simulink model "meat_1024pt_bee2_sign"  (Simulink 6.2)
settings: Solver=ode45  StartTime=0.0  StopTime=60000  RelTol=1e-3
undefined symbols (not defined in the file): BEE2_usr, bit_rev, pfb_coeff_gen_calc
libraries: xbsIndex_r3 x1079, casper_library x94, xps_library x27
(part 2 of 8)

== system meat_1024pt_bee2_sign/fft ==
  sync : Inport  Port=1  LatchInput=off
  shift : Inport  Port=2  LatchInput=off
  pol0 : Inport  Port=3  LatchInput=off
  pol1 : Inport  Port=4  LatchInput=off
  fft_biplex0 : Subsystem  AncestorBlock=casper_library/FFTs/fft_biplex  mask(fft_biplex){FFTSize=10, BitWidth=18, quantization=Truncate, overflow=Wrap, add_latency=3, mult_latency=4, bram_latency=3}
      mask prompts: FFTSize "Size of FFT: (2^? pnts)"; BitWidth "Bitwidth: (Max Efficiency at 18 bits)"; quantization "Quantization Behavior"; overflow "Overflow Behavior"; add_latency "Add Latency"; mult_latency "Mult Latency"; bram_latency "BRAM Latency"
      mask init:
      | fft_biplex_init(gcb,...
      |     'FFTSize', FFTSize,...
      |     'BitWidth', BitWidth,...
      |     'quantization', quantization,...
      |     'overflow', overflow,...
      |     'add_latency', add_latency,...
      |     'mult_latency', mult_latency,...
      |     'bram_latency', bram_latency);
      settings: AttributesFormatString=FFTSize=10, BitWidth=18
      mask StyleString: edit,edit,popup(Truncate|Round  (unbiased: +/- Inf)|Round  (unbiased: Even Values)),popup(Wrap|Saturate|Error),edit,edit,edit
  sync_out : Outport
  out0 : Outport  Port=2
  out1 : Outport  Port=3
  wires:
  pol0/1 -> fft_biplex0/1(pol1)
  pol1/1 -> fft_biplex0/2(pol2)
  shift/1 -> fft_biplex0/4(shift)
  sync/1 -> fft_biplex0/3(sync)
  fft_biplex0/1(pol1_out) -> out0/1
  fft_biplex0/2(pol2_out) -> out1/1
  fft_biplex0/4(sync_out) -> sync_out/1

== system meat_1024pt_bee2_sign/pfb_fir ==
  sync : Inport  Port=1  LatchInput=off
  pol1_in1 : Inport  Port=2  LatchInput=off
  pol2_in1 : Inport  Port=3  LatchInput=off
  pol1_in1_first_tap : Subsystem  AncestorBlock=casper_library/PFBs/first_tap  mask(first_tap){nput=0, PFBSize=10, CoeffBitWidth=8, TotalTaps=4, BitWidthIn=8, CoeffDistMem=1, WindowType=hamming, mult_latency=3, bram_latency=3, n_inputs=0, fwidth=1}
      mask prompts: nput "This is input number:"; PFBSize "Size of PFB: (2^? pnts)"; CoeffBitWidth "Bitwidth of Coefficients:"; TotalTaps "Total Number of Taps:"; BitWidthIn "Input Bitwidth:"; CoeffDistMem "Implement Coeff Gen in Distributed Memory:"; WindowType "Windowing Function:"; mult_latency "Mult Latency"; bram_latency "BRAM Latency"; n_inputs "Number of Simultaneous Inputs: (2^?)"; fwidth "Bit Width (normal=1)"
      mask init:
      | first_tap_init(gcb,...
      |     'nput', nput,...
      |     'PFBSize', PFBSize,...
      |     'CoeffBitWidth', CoeffBitWidth,...
      |     'TotalTaps', TotalTaps,...
      |     'BitWidthIn', BitWidthIn,...
      |     'CoeffDistMem', CoeffDistMem,...
      |     'WindowType', WindowType,...
      |     'mult_latency', mult_latency,...
      |     'bram_latency', bram_latency,...
      |     'n_inputs', n_inputs,...
      |     'fwidth', fwidth);
      settings: AttributesFormatString=input=0, taps=4
      mask StyleString: edit,edit,edit,edit,edit,edit,popup(bartlett|barthannwin|blackman|blackmanharris|bohamwin|chebwin|flattopwin|gausswin|hamming|hann|kaiser|nuttallwin|parzenwin|rectwin|tukeywin|triang),edit,edit,edit,edit
  pol1_in1_last_tap : Subsystem  AncestorBlock=casper_library/PFBs/last_tap  mask(last_tap){TotalTaps=4, BitWidthIn=8, BitWidthOut=18, CoeffBitWidth=8, add_latency=2, mult_latency=3, quantization=Truncate}
      mask prompts: TotalTaps "Total Number of Taps:"; BitWidthIn "Input Bitwidth:"; BitWidthOut "Output Bitwidth:"; CoeffBitWidth "Coeff Bitwidth:"; add_latency "Add Latency"; mult_latency "Mult Latency"; quantization "Quantization Behavior"
      mask init:
      | last_tap_init(gcb,...
      |     'TotalTaps', TotalTaps,...
      |     'BitWidthIn', BitWidthIn,...
      |     'BitWidthOut', BitWidthOut,...
      |     'CoeffBitWidth', CoeffBitWidth,...
      |     'add_latency', add_latency,...
      |     'mult_latency', mult_latency,...
      |     'quantization', quantization);
      settings: AttributesFormatString=taps=4
      mask StyleString: edit,edit,edit,edit,edit,edit,popup(Truncate|Round  (unbiased: +/- Inf)|Round  (unbiased: Even Values))
  pol1_in1_tap2 : casper_library/PFBs/tap
      link override delay/delay_bram/Constant2: equ=P=C
      link override sync_delay/Constant: equ=P=C
      link override sync_delay/Constant1: equ=P=C
      link override sync_delay/Constant2: equ=P=C
      link override sync_delay/Constant3: equ=P=C
  pol1_in1_tap3 : casper_library/PFBs/tap
      link override delay/delay_bram/Constant2: equ=P=C
      link override sync_delay/Constant: equ=P=C
      link override sync_delay/Constant1: equ=P=C
      link override sync_delay/Constant2: equ=P=C
      link override sync_delay/Constant3: equ=P=C
  pol2_in1_first_tap : Subsystem  AncestorBlock=casper_library/PFBs/first_tap  mask(first_tap){nput=0, PFBSize=10, CoeffBitWidth=8, TotalTaps=4, BitWidthIn=8, CoeffDistMem=1, WindowType=hamming, mult_latency=3, bram_latency=3, n_inputs=0, fwidth=1}
      mask prompts: nput "This is input number:"; PFBSize "Size of PFB: (2^? pnts)"; CoeffBitWidth "Bitwidth of Coefficients:"; TotalTaps "Total Number of Taps:"; BitWidthIn "Input Bitwidth:"; CoeffDistMem "Implement Coeff Gen in Distributed Memory:"; WindowType "Windowing Function:"; mult_latency "Mult Latency"; bram_latency "BRAM Latency"; n_inputs "Number of Simultaneous Inputs: (2^?)"; fwidth "Bit Width (normal=1)"
      mask init: same as meat_1024pt_bee2_sign/pfb_fir/pol1_in1_first_tap
      settings: AttributesFormatString=input=0, taps=4
      mask StyleString: edit,edit,edit,edit,edit,edit,popup(bartlett|barthannwin|blackman|blackmanharris|bohamwin|chebwin|flattopwin|gausswin|hamming|hann|kaiser|nuttallwin|parzenwin|rectwin|tukeywin|triang),edit,edit,edit,edit
  pol2_in1_last_tap : Subsystem  AncestorBlock=casper_library/PFBs/last_tap  mask(last_tap){TotalTaps=4, BitWidthIn=8, BitWidthOut=18, CoeffBitWidth=8, add_latency=2, mult_latency=3, quantization=Truncate}
      mask prompts: TotalTaps "Total Number of Taps:"; BitWidthIn "Input Bitwidth:"; BitWidthOut "Output Bitwidth:"; CoeffBitWidth "Coeff Bitwidth:"; add_latency "Add Latency"; mult_latency "Mult Latency"; quantization "Quantization Behavior"
      mask init: same as meat_1024pt_bee2_sign/pfb_fir/pol1_in1_last_tap
      settings: AttributesFormatString=taps=4
      mask StyleString: edit,edit,edit,edit,edit,edit,popup(Truncate|Round  (unbiased: +/- Inf)|Round  (unbiased: Even Values))
  pol2_in1_tap2 : casper_library/PFBs/tap
      link override delay/delay_bram/Constant2: equ=P=C
      link override sync_delay/Constant: equ=P=C
      link override sync_delay/Constant1: equ=P=C
      link override sync_delay/Constant2: equ=P=C
      link override sync_delay/Constant3: equ=P=C
  pol2_in1_tap3 : casper_library/PFBs/tap
      link override delay/delay_bram/Constant2: equ=P=C
      link override sync_delay/Constant: equ=P=C
      link override sync_delay/Constant1: equ=P=C
      link override sync_delay/Constant2: equ=P=C
      link override sync_delay/Constant3: equ=P=C
  sync_out : Outport
  pol1_out1 : Outport  Port=2
  pol2_out1 : Outport  Port=3
  wires:
  pol1_in1/1 -> pol1_in1_first_tap/1(din)
  sync/1 -> pol1_in1_first_tap/2(sync), pol2_in1_first_tap/2(sync)
  pol1_in1_first_tap/1(dout) -> pol1_in1_tap2/1
  pol1_in1_first_tap/2(sync_out) -> pol1_in1_tap2/2
  pol1_in1_first_tap/3(coeff_out) -> pol1_in1_tap2/3
  pol1_in1_first_tap/4(taps_out) -> pol1_in1_tap2/4
  pol1_in1_tap2/1 -> pol1_in1_tap3/1
  pol1_in1_tap2/2 -> pol1_in1_tap3/2
  pol1_in1_tap2/3 -> pol1_in1_tap3/3
  pol1_in1_tap2/4 -> pol1_in1_tap3/4
  pol1_in1_tap3/1 -> pol1_in1_last_tap/1(din)
  pol1_in1_tap3/2 -> pol1_in1_last_tap/2(sync)
  pol1_in1_tap3/3 -> pol1_in1_last_tap/3(coeff)
  pol1_in1_tap3/4 -> pol1_in1_last_tap/4(taps)
  pol1_in1_last_tap/1(dout) -> pol1_out1/1
  pol1_in1_last_tap/2(sync_out) -> sync_out/1
  pol2_in1/1 -> pol2_in1_first_tap/1(din)
  pol2_in1_first_tap/1(dout) -> pol2_in1_tap2/1
  pol2_in1_first_tap/2(sync_out) -> pol2_in1_tap2/2
  pol2_in1_first_tap/3(coeff_out) -> pol2_in1_tap2/3
  pol2_in1_first_tap/4(taps_out) -> pol2_in1_tap2/4
  pol2_in1_tap2/1 -> pol2_in1_tap3/1
  pol2_in1_tap2/2 -> pol2_in1_tap3/2
  pol2_in1_tap2/3 -> pol2_in1_tap3/3
  pol2_in1_tap2/4 -> pol2_in1_tap3/4
  pol2_in1_tap3/1 -> pol2_in1_last_tap/1(din)
  pol2_in1_tap3/2 -> pol2_in1_last_tap/2(sync)
  pol2_in1_tap3/3 -> pol2_in1_last_tap/3(coeff)
  pol2_in1_tap3/4 -> pol2_in1_last_tap/4(taps)
  pol2_in1_last_tap/1(dout) -> pol2_out1/1

== system meat_1024pt_bee2_sign/pol1_kurt1 ==
  note: Input unsigned 24-bits, b.p. at 23
  note: Output unsigned 24-bits, b.p. at 23
  note: Unsigned, 18-bits, b.p. at 12
  coeff : Inport  Orientation=down  Port=1  LatchInput=off
  data_in : Inport  Port=2  LatchInput=off
  Convert : xbsIndex_r3/Convert  arith_type=Unsigned  n_bits=32  bin_pt=31  quantization=Truncate  overflow=Wrap  latency=1  explicit_period=off  period=1  dbl_ovrd=off  show_param=off  inserted_by_tool=off  pipeline=off
      settings: xl_area=[0, 0, 0, 0, 0, 0, 0]
  mult_coeff_fft_real : xbsIndex_r3/Mult  precision=Full  arith_type="Signed  (2's comp)"  n_bits=24  bin_pt=23  quantization=Truncate  overflow=Wrap  latency=5  explicit_period=off  period=1  en=off  dbl_ovrd=off  show_param=on  mult_type=Parallel  oversample=2  use_embedded=on  pipeline=on  use_rpm=on  placement_style=Rectangular Shape  gen_core=off
      settings: xl_area=[0, 0, 0, 0, 0, 0, 0]
  data_out : Outport
  wires:
  Convert/1 -> data_out/1
  data_in/1 -> mult_coeff_fft_real/2
  coeff/1 -> mult_coeff_fft_real/1
  mult_coeff_fft_real/1 -> Convert/1

== system meat_1024pt_bee2_sign/pol2_kurt1 ==
  note: Unsigned, 18-bits, b.p. at 12
  note: Output unsigned 24-bits, b.p. at 23
  note: Input unsigned 24-bits, b.p. at 23
  coeff : Inport  Orientation=down  Port=1  LatchInput=off
  data_in : Inport  Port=2  LatchInput=off
  Convert : xbsIndex_r3/Convert  arith_type=Unsigned  n_bits=32  bin_pt=31  quantization=Truncate  overflow=Wrap  latency=1  explicit_period=off  period=1  dbl_ovrd=off  show_param=off  inserted_by_tool=off  pipeline=off
      settings: xl_area=[0, 0, 0, 0, 0, 0, 0]
  mult_coeff_fft_real : xbsIndex_r3/Mult  precision=Full  arith_type="Signed  (2's comp)"  n_bits=24  bin_pt=23  quantization=Truncate  overflow=Wrap  latency=5  explicit_period=off  period=1  en=off  dbl_ovrd=off  show_param=on  mult_type=Parallel  oversample=2  use_embedded=on  pipeline=on  use_rpm=on  placement_style=Rectangular Shape  gen_core=off
      settings: xl_area=[0, 0, 0, 0, 0, 0, 0]
  data_out : Outport
  wires:
  Convert/1 -> data_out/1
  mult_coeff_fft_real/1 -> Convert/1
  coeff/1 -> mult_coeff_fft_real/1
  data_in/1 -> mult_coeff_fft_real/2

== system meat_1024pt_bee2_sign/signed_bitselect ==
  bitselect : Inport  Port=1  LatchInput=off
  data_in : Inport  Port=2  LatchInput=off
  0-6_inclusive : xbsIndex_r3/Slice  mode=Lower Bit Location + Width  nbits=7  bit1=0  base1=MSB of Input  bit0=0  base0=LSB of Input  boolean_output=off  explicit_period=off  period=1  dbl_ovrd=off
  14-20_inclusive : xbsIndex_r3/Slice  mode=Lower Bit Location + Width  nbits=7  bit1=0  base1=MSB of Input  bit0=14  base0=LSB of Input  boolean_output=off  explicit_period=off  period=1  dbl_ovrd=off
  21-27_inclusive : xbsIndex_r3/Slice  mode=Lower Bit Location + Width  nbits=7  bit1=0  base1=MSB of Input  bit0=7  base0=LSB of Input  boolean_output=off  explicit_period=off  period=1  dbl_ovrd=off
  28-34_inclusive : xbsIndex_r3/Slice  mode=Lower Bit Location + Width  nbits=7  bit1=0  base1=MSB of Input  bit0=7  base0=LSB of Input  boolean_output=off  explicit_period=off  period=1  dbl_ovrd=off
  35-41_inclusive : xbsIndex_r3/Slice  mode=Lower Bit Location + Width  nbits=7  bit1=0  base1=MSB of Input  bit0=7  base0=LSB of Input  boolean_output=off  explicit_period=off  period=1  dbl_ovrd=off
  40-47_inclusive : xbsIndex_r3/Slice  mode=Lower Bit Location + Width  nbits=7  bit1=0  base1=MSB of Input  bit0=7  base0=LSB of Input  boolean_output=off  explicit_period=off  period=1  dbl_ovrd=off
  7-13_inclusive : xbsIndex_r3/Slice  mode=Lower Bit Location + Width  nbits=7  bit1=0  base1=MSB of Input  bit0=7  base0=LSB of Input  boolean_output=off  explicit_period=off  period=1  dbl_ovrd=off
  Concat{,1..5} (6 alike) : xbsIndex_r3/Concat  num_inputs=2  explicit_period=off  period=1  dbl_ovrd=off
  Mux : xbsIndex_r3/Mux  inputs=7  precision=Full  arith_type="Signed  (2's comp)"  n_bits=8  bin_pt=2  quantization=Truncate  overflow=Wrap  latency=0  explicit_period=off  period=1  en=off  dbl_ovrd=off  show_param=off  mux_type=off  use_rpm=off  gen_core=off
      settings: xl_area=[0, 0, 0, 0, 0, 0, 0]
  sign_bit : xbsIndex_r3/Slice  mode=Upper Bit Location + Width  nbits=1  bit1=0  base1=MSB of Input  bit0=0  base0=LSB of Input  boolean_output=off  explicit_period=off  period=1  dbl_ovrd=off
  data_out : Outport
  wires:
  Mux/1 -> data_out/1
  bitselect/1 -> Mux/1
  0-6_inclusive/1 -> Concat/2
  7-13_inclusive/1 -> Concat1/2
  14-20_inclusive/1 -> Concat2/2
  21-27_inclusive/1 -> Concat3/2
  28-34_inclusive/1 -> Concat4/2
  35-41_inclusive/1 -> Concat5/2
  sign_bit/1 -> Concat/1, Concat1/1, Concat2/1, Concat3/1, Concat4/1, Concat5/1
  data_in/1 -> sign_bit/1, 0-6_inclusive/1, 7-13_inclusive/1, 14-20_inclusive/1, 21-27_inclusive/1, 28-34_inclusive/1, 35-41_inclusive/1, 40-47_inclusive/1
  Concat/1 -> Mux/2
  Concat1/1 -> Mux/3
  Concat2/1 -> Mux/4
  Concat3/1 -> Mux/5
  Concat4/1 -> Mux/6
  Concat5/1 -> Mux/7
  40-47_inclusive/1 -> Mux/8

== system meat_1024pt_bee2_sign/signed_bitselect_1 ==
  bitselect : Inport  Port=1  LatchInput=off
  data_in : Inport  Port=2  LatchInput=off
  0-6_inclusive : xbsIndex_r3/Slice  mode=Lower Bit Location + Width  nbits=7  bit1=0  base1=MSB of Input  bit0=0  base0=LSB of Input  boolean_output=off  explicit_period=off  period=1  dbl_ovrd=off
  14-20_inclusive : xbsIndex_r3/Slice  mode=Lower Bit Location + Width  nbits=7  bit1=0  base1=MSB of Input  bit0=14  base0=LSB of Input  boolean_output=off  explicit_period=off  period=1  dbl_ovrd=off
  21-27_inclusive : xbsIndex_r3/Slice  mode=Lower Bit Location + Width  nbits=7  bit1=0  base1=MSB of Input  bit0=7  base0=LSB of Input  boolean_output=off  explicit_period=off  period=1  dbl_ovrd=off
  28-34_inclusive : xbsIndex_r3/Slice  mode=Lower Bit Location + Width  nbits=7  bit1=0  base1=MSB of Input  bit0=7  base0=LSB of Input  boolean_output=off  explicit_period=off  period=1  dbl_ovrd=off
  35-41_inclusive : xbsIndex_r3/Slice  mode=Lower Bit Location + Width  nbits=7  bit1=0  base1=MSB of Input  bit0=7  base0=LSB of Input  boolean_output=off  explicit_period=off  period=1  dbl_ovrd=off
  40-47_inclusive : xbsIndex_r3/Slice  mode=Lower Bit Location + Width  nbits=7  bit1=0  base1=MSB of Input  bit0=7  base0=LSB of Input  boolean_output=off  explicit_period=off  period=1  dbl_ovrd=off
  7-13_inclusive : xbsIndex_r3/Slice  mode=Lower Bit Location + Width  nbits=7  bit1=0  base1=MSB of Input  bit0=7  base0=LSB of Input  boolean_output=off  explicit_period=off  period=1  dbl_ovrd=off
  Concat{,1..5} (6 alike) : xbsIndex_r3/Concat  num_inputs=2  explicit_period=off  period=1  dbl_ovrd=off
  Mux : xbsIndex_r3/Mux  inputs=7  precision=Full  arith_type="Signed  (2's comp)"  n_bits=8  bin_pt=2  quantization=Truncate  overflow=Wrap  latency=0  explicit_period=off  period=1  en=off  dbl_ovrd=off  show_param=off  mux_type=off  use_rpm=off  gen_core=off
      settings: xl_area=[0, 0, 0, 0, 0, 0, 0]
  sign_bit : xbsIndex_r3/Slice  mode=Upper Bit Location + Width  nbits=1  bit1=0  base1=MSB of Input  bit0=0  base0=LSB of Input  boolean_output=off  explicit_period=off  period=1  dbl_ovrd=off
  data_out : Outport
  wires:
  40-47_inclusive/1 -> Mux/8
  Concat5/1 -> Mux/7
  Concat4/1 -> Mux/6
  Concat3/1 -> Mux/5
  Concat2/1 -> Mux/4
  Concat1/1 -> Mux/3
  Concat/1 -> Mux/2
  data_in/1 -> 40-47_inclusive/1, 35-41_inclusive/1, 28-34_inclusive/1, 21-27_inclusive/1, 14-20_inclusive/1, 7-13_inclusive/1, 0-6_inclusive/1, sign_bit/1
  sign_bit/1 -> Concat5/1, Concat4/1, Concat3/1, Concat2/1, Concat1/1, Concat/1
  35-41_inclusive/1 -> Concat5/2
  28-34_inclusive/1 -> Concat4/2
  21-27_inclusive/1 -> Concat3/2
  14-20_inclusive/1 -> Concat2/2
  7-13_inclusive/1 -> Concat1/2
  0-6_inclusive/1 -> Concat/2
  bitselect/1 -> Mux/1
  Mux/1 -> data_out/1

== system meat_1024pt_bee2_sign/signed_scale2 ==
  note: Input signed 24-bits, b.p. at 23
  note: Output signed 24-bits, b.p. at 23
  note: Unsigned, 18-bits, b.p. at 12
  coeff : Inport  Orientation=down  Port=1  LatchInput=off
  data_in : Inport  Port=2  LatchInput=off
  Convert : xbsIndex_r3/Convert  arith_type="Signed  (2's comp)"  n_bits=32  bin_pt=31  quantization=Truncate  overflow=Wrap  latency=1  explicit_period=off  period=1  dbl_ovrd=off  show_param=off  inserted_by_tool=off  pipeline=off
      settings: xl_area=[0, 0, 0, 0, 0, 0, 0]
  mult_coeff_fft_real : xbsIndex_r3/Mult  precision=Full  arith_type="Signed  (2's comp)"  n_bits=24  bin_pt=23  quantization=Truncate  overflow=Wrap  latency=5  explicit_period=off  period=1  en=off  dbl_ovrd=off  show_param=on  mult_type=Parallel  oversample=2  use_embedded=on  pipeline=on  use_rpm=on  placement_style=Rectangular Shape  gen_core=off
      settings: xl_area=[0, 0, 0, 0, 0, 0, 0]
  data_out : Outport
  wires:
  data_in/1 -> mult_coeff_fft_real/2
  coeff/1 -> mult_coeff_fft_real/1
  mult_coeff_fft_real/1 -> Convert/1
  Convert/1 -> data_out/1

== system meat_1024pt_bee2_sign/signed_scale3 ==
  note: Unsigned, 18-bits, b.p. at 12
  note: Output signed 24-bits, b.p. at 23
  note: Input signed 24-bits, b.p. at 23
  coeff : Inport  Orientation=down  Port=1  LatchInput=off
  data_in : Inport  Port=2  LatchInput=off
  Convert : xbsIndex_r3/Convert  arith_type="Signed  (2's comp)"  n_bits=32  bin_pt=31  quantization=Truncate  overflow=Wrap  latency=1  explicit_period=off  period=1  dbl_ovrd=off  show_param=off  inserted_by_tool=off  pipeline=off
      settings: xl_area=[0, 0, 0, 0, 0, 0, 0]
  mult_coeff_fft_real : xbsIndex_r3/Mult  precision=Full  arith_type="Signed  (2's comp)"  n_bits=24  bin_pt=23  quantization=Truncate  overflow=Wrap  latency=5  explicit_period=off  period=1  en=off  dbl_ovrd=off  show_param=on  mult_type=Parallel  oversample=2  use_embedded=on  pipeline=on  use_rpm=on  placement_style=Rectangular Shape  gen_core=off
      settings: xl_area=[0, 0, 0, 0, 0, 0, 0]
  data_out : Outport
  wires:
  mult_coeff_fft_real/1 -> Convert/1
  coeff/1 -> mult_coeff_fft_real/1
  data_in/1 -> mult_coeff_fft_real/2
  Convert/1 -> data_out/1

== system meat_1024pt_bee2_sign/sync_generator ==
  period : Inport  Port=1  LatchInput=off
  reset : Inport  Port=2  LatchInput=off
  Convert : xbsIndex_r3/Convert  arith_type=Boolean  n_bits=8  bin_pt=6  quantization=Truncate  overflow=Wrap  latency=1  explicit_period=off  period=1  dbl_ovrd=off  show_param=off  inserted_by_tool=off  pipeline=off
      settings: xl_area=[0, 0, 0, 0, 0, 0, 0]
  Counter : xbsIndex_r3/Counter  cnt_type=Free Running  n_bits=32  bin_pt=0  arith_type=Unsigned  start_count=1  cnt_to=Inf  cnt_by_val=1  operation=Up  explicit_period=on  period=1  load_pin=off  rst=on  en=off  dbl_ovrd=off  show_param=off  use_rpm=on  gen_core=off
      settings: xl_area=[0, 0, 0, 0, 0, 0, 0]
  Logical : xbsIndex_r3/Logical  logical_function=OR  inputs=2  precision=Full  arith_type=Unsigned  n_bits=8  bin_pt=2  align_bp=on  latency=0  explicit_period=off  period=1  en=off  dbl_ovrd=off  show_param=off
      settings: xl_area=[0, 0, 0, 0, 0, 0, 0]
  Relational : xbsIndex_r3/Relational  mode=a>=b  latency=1  explicit_period=off  period=1  en=off  dbl_ovrd=off  show_param=off
      settings: xl_area=[0, 0, 0, 0, 0, 0, 0]
  cns : xbsIndex_r3/Constant  const=4  equ=P=C  arith_type=Unsigned  n_bits=3  bin_pt=0  opselect=C  inp2=PCIN>>17  opr=+  inp1=P  carry=CIN  iostate=0  explicit_period=off  period=1  dbl_ovrd=off
  period_sub : xbsIndex_r3/AddSub  mode=Subtraction  precision=User Defined  arith_type=Unsigned  n_bits=32  bin_pt=0  quantization=Truncate  overflow=Wrap  latency=0  explicit_period=off  period=1  use_carryin=off  use_carryout=off  en=off  dbl_ovrd=off  show_param=off  use_core=on  pipeline=off  use_rpm=on  gen_core=off
      settings: xl_area=[0, 0, 0, 0, 0, 0, 0]
  posedge : casper_library/Misc/posedge  Tag=Rising Edge Detector
  sync : Outport
  wires:
  Counter/1 -> Relational/1
  Relational/1 -> Convert/1
  Convert/1 -> Logical/2
  Logical/1 -> Counter/1, posedge/1
  reset/1 -> Logical/1
  period/1 -> period_sub/1
  period_sub/1 -> Relational/2
  cns/1 -> period_sub/2
  posedge/1 -> sync/1

== system meat_1024pt_bee2_sign/uncram_crossterms ==
  In : Inport  Port=1  LatchInput=off
  Reinterp1 : xbsIndex_r3/Reinterpret  force_arith_type=on  arith_type="Signed  (2's comp)"  force_bin_pt=on  bin_pt=31  force_valid=on
  Reinterp2 : xbsIndex_r3/Reinterpret  force_arith_type=on  arith_type="Signed  (2's comp)"  force_bin_pt=on  bin_pt=31  force_valid=on
  Slice1 : xbsIndex_r3/Slice  mode=Upper Bit Location + Width  nbits=48  bit1=0  base1=MSB of Input  bit0=0  base0=LSB of Input  boolean_output=off  explicit_period=off  period=1  dbl_ovrd=off
  Slice2 : xbsIndex_r3/Slice  mode=Upper Bit Location + Width  nbits=48  bit1=-48  base1=MSB of Input  bit0=0  base0=LSB of Input  boolean_output=off  explicit_period=off  period=1  dbl_ovrd=off
  Out1 : Outport
  Out2 : Outport  Port=2
  wires:
  In/1 -> Slice1/1, Slice2/1
  Slice1/1 -> Reinterp1/1
  Reinterp1/1 -> Out1/1
  Slice2/1 -> Reinterp2/1
  Reinterp2/1 -> Out2/1

== system meat_1024pt_bee2_sign/uncram_powers ==
  In : Inport  Port=1  LatchInput=off
  Reinterp1 : xbsIndex_r3/Reinterpret  force_arith_type=on  arith_type=Unsigned  force_bin_pt=on  bin_pt=31  force_valid=on
  Reinterp2 : xbsIndex_r3/Reinterpret  force_arith_type=on  arith_type=Unsigned  force_bin_pt=on  bin_pt=31  force_valid=on
  Slice1 : xbsIndex_r3/Slice  mode=Upper Bit Location + Width  nbits=48  bit1=0  base1=MSB of Input  bit0=0  base0=LSB of Input  boolean_output=off  explicit_period=off  period=1  dbl_ovrd=off
  Slice2 : xbsIndex_r3/Slice  mode=Upper Bit Location + Width  nbits=48  bit1=-48  base1=MSB of Input  bit0=0  base0=LSB of Input  boolean_output=off  explicit_period=off  period=1  dbl_ovrd=off
  Out1 : Outport
  Out2 : Outport  Port=2
  wires:
  In/1 -> Slice1/1, Slice2/1
  Slice1/1 -> Reinterp1/1
  Reinterp1/1 -> Out1/1
  Slice2/1 -> Reinterp2/1
  Reinterp2/1 -> Out2/1

== system meat_1024pt_bee2_sign/uncram_powers1 ==
  In : Inport  Port=1  LatchInput=off
  Reinterp1 : xbsIndex_r3/Reinterpret  force_arith_type=on  arith_type=Unsigned  force_bin_pt=on  bin_pt=46  force_valid=on
  Reinterp2 : xbsIndex_r3/Reinterpret  force_arith_type=on  arith_type=Unsigned  force_bin_pt=on  bin_pt=46  force_valid=on
  Slice1 : xbsIndex_r3/Slice  mode=Upper Bit Location + Width  nbits=64  bit1=0  base1=MSB of Input  bit0=0  base0=LSB of Input  boolean_output=off  explicit_period=off  period=1  dbl_ovrd=off
  Slice2 : xbsIndex_r3/Slice  mode=Upper Bit Location + Width  nbits=64  bit1=-64  base1=MSB of Input  bit0=0  base0=LSB of Input  boolean_output=off  explicit_period=off  period=1  dbl_ovrd=off
  Out1 : Outport
  Out2 : Outport  Port=2
  wires:
  In/1 -> Slice1/1, Slice2/1
  Slice1/1 -> Reinterp1/1
  Reinterp1/1 -> Out1/1
  Slice2/1 -> Reinterp2/1
  Reinterp2/1 -> Out2/1

== system meat_1024pt_bee2_sign/unsigned_bitselect_1 ==
  bitselect : Inport  Port=1  LatchInput=off
  data_in : Inport  Port=2  LatchInput=off
  mux_bitselect : xbsIndex_r3/Mux  inputs=6  precision=Full  arith_type="Signed  (2's comp)"  n_bits=8  bin_pt=2  quantization=Truncate  overflow=Wrap  latency=1  explicit_period=off  period=1  en=off  dbl_ovrd=off  show_param=off  mux_type=off  use_rpm=off  gen_core=off
      settings: xl_area=[0, 0, 0, 0, 0, 0, 0]
  reint_bp_0 : xbsIndex_r3/Reinterpret  force_arith_type=on  arith_type=Unsigned  force_bin_pt=on  bin_pt=0  force_valid=on
  slc_bitselect_1 : xbsIndex_r3/Slice  mode=Lower Bit Location + Width  nbits=8  bit1=0  base1=MSB of Input  bit0=0  base0=LSB of Input  boolean_output=off  explicit_period=off  period=1  dbl_ovrd=off
  slc_bitselect_2 : xbsIndex_r3/Slice  mode=Lower Bit Location + Width  nbits=8  bit1=0  base1=MSB of Input  bit0=8  base0=LSB of Input  boolean_output=off  explicit_period=off  period=1  dbl_ovrd=off
  slc_bitselect_3 : xbsIndex_r3/Slice  mode=Lower Bit Location + Width  nbits=8  bit1=0  base1=MSB of Input  bit0=16  base0=LSB of Input  boolean_output=off  explicit_period=off  period=1  dbl_ovrd=off
  slc_bitselect_4 : xbsIndex_r3/Slice  mode=Lower Bit Location + Width  nbits=8  bit1=0  base1=MSB of Input  bit0=24  base0=LSB of Input  boolean_output=off  explicit_period=off  period=1  dbl_ovrd=off
  slc_bitselect_5 : xbsIndex_r3/Slice  mode=Lower Bit Location + Width  nbits=8  bit1=0  base1=MSB of Input  bit0=32  base0=LSB of Input  boolean_output=off  explicit_period=off  period=1  dbl_ovrd=off
  slc_bitselect_6 : xbsIndex_r3/Slice  mode=Lower Bit Location + Width  nbits=8  bit1=0  base1=MSB of Input  bit0=40  base0=LSB of Input  boolean_output=off  explicit_period=off  period=1  dbl_ovrd=off
  data_out : Outport
  wires:
  reint_bp_0/1 -> slc_bitselect_1/1, slc_bitselect_2/1, slc_bitselect_3/1, slc_bitselect_4/1, slc_bitselect_5/1, slc_bitselect_6/1
  mux_bitselect/1 -> data_out/1
  bitselect/1 -> mux_bitselect/1
  data_in/1 -> reint_bp_0/1
  slc_bitselect_4/1 -> mux_bitselect/5
  slc_bitselect_3/1 -> mux_bitselect/4
  slc_bitselect_2/1 -> mux_bitselect/3
  slc_bitselect_1/1 -> mux_bitselect/2
  slc_bitselect_6/1 -> mux_bitselect/7
  slc_bitselect_5/1 -> mux_bitselect/6

== system meat_1024pt_bee2_sign/unsigned_bitselect_2 ==
  bitselect : Inport  Port=1  LatchInput=off
  data_in : Inport  Port=2  LatchInput=off
  mux_bitselect : xbsIndex_r3/Mux  inputs=7  precision=Full  arith_type="Signed  (2's comp)"  n_bits=8  bin_pt=2  quantization=Truncate  overflow=Wrap  latency=1  explicit_period=off  period=1  en=off  dbl_ovrd=off  show_param=off  mux_type=off  use_rpm=off  gen_core=off
      settings: xl_area=[0, 0, 0, 0, 0, 0, 0]
  reint_bp_0 : xbsIndex_r3/Reinterpret  force_arith_type=on  arith_type=Unsigned  force_bin_pt=on  bin_pt=0  force_valid=on
  slc_bitselect_1 : xbsIndex_r3/Slice  mode=Lower Bit Location + Width  nbits=16  bit1=0  base1=MSB of Input  bit0=0  base0=LSB of Input  boolean_output=off  explicit_period=off  period=1  dbl_ovrd=off
  slc_bitselect_2 : xbsIndex_r3/Slice  mode=Lower Bit Location + Width  nbits=16  bit1=0  base1=MSB of Input  bit0=8  base0=LSB of Input  boolean_output=off  explicit_period=off  period=1  dbl_ovrd=off
  slc_bitselect_3 : xbsIndex_r3/Slice  mode=Lower Bit Location + Width  nbits=16  bit1=0  base1=MSB of Input  bit0=16  base0=LSB of Input  boolean_output=off  explicit_period=off  period=1  dbl_ovrd=off
  slc_bitselect_4 : xbsIndex_r3/Slice  mode=Lower Bit Location + Width  nbits=16  bit1=0  base1=MSB of Input  bit0=24  base0=LSB of Input  boolean_output=off  explicit_period=off  period=1  dbl_ovrd=off
  slc_bitselect_5 : xbsIndex_r3/Slice  mode=Lower Bit Location + Width  nbits=16  bit1=0  base1=MSB of Input  bit0=32  base0=LSB of Input  boolean_output=off  explicit_period=off  period=1  dbl_ovrd=off
  slc_bitselect_6 : xbsIndex_r3/Slice  mode=Lower Bit Location + Width  nbits=16  bit1=0  base1=MSB of Input  bit0=40  base0=LSB of Input  boolean_output=off  explicit_period=off  period=1  dbl_ovrd=off
  slc_bitselect_7 : xbsIndex_r3/Slice  mode=Lower Bit Location + Width  nbits=16  bit1=0  base1=MSB of Input  bit0=48  base0=LSB of Input  boolean_output=off  explicit_period=off  period=1  dbl_ovrd=off
  data_out : Outport
  wires:
  slc_bitselect_6/1 -> mux_bitselect/7
  slc_bitselect_7/1 -> mux_bitselect/8
  slc_bitselect_5/1 -> mux_bitselect/6
  reint_bp_0/1 -> slc_bitselect_1/1, slc_bitselect_2/1, slc_bitselect_7/1, slc_bitselect_6/1, slc_bitselect_5/1, slc_bitselect_4/1, slc_bitselect_3/1
  mux_bitselect/1 -> data_out/1
  bitselect/1 -> mux_bitselect/1
  data_in/1 -> reint_bp_0/1
  slc_bitselect_4/1 -> mux_bitselect/5
  slc_bitselect_3/1 -> mux_bitselect/4
  slc_bitselect_2/1 -> mux_bitselect/3
  slc_bitselect_1/1 -> mux_bitselect/2

== system meat_1024pt_bee2_sign/unsigned_bitselect_3 ==
  bitselect : Inport  Port=1  LatchInput=off
  data_in : Inport  Port=2  LatchInput=off
  mux_bitselect : xbsIndex_r3/Mux  inputs=7  precision=Full  arith_type="Signed  (2's comp)"  n_bits=8  bin_pt=2  quantization=Truncate  overflow=Wrap  latency=1  explicit_period=off  period=1  en=off  dbl_ovrd=off  show_param=off  mux_type=off  use_rpm=off  gen_core=off
      settings: xl_area=[0, 0, 0, 0, 0, 0, 0]
  reint_bp_0 : xbsIndex_r3/Reinterpret  force_arith_type=on  arith_type=Unsigned  force_bin_pt=on  bin_pt=0  force_valid=on
  slc_bitselect_1 : xbsIndex_r3/Slice  mode=Lower Bit Location + Width  nbits=16  bit1=0  base1=MSB of Input  bit0=0  base0=LSB of Input  boolean_output=off  explicit_period=off  period=1  dbl_ovrd=off
  slc_bitselect_2 : xbsIndex_r3/Slice  mode=Lower Bit Location + Width  nbits=16  bit1=0  base1=MSB of Input  bit0=8  base0=LSB of Input  boolean_output=off  explicit_period=off  period=1  dbl_ovrd=off
  slc_bitselect_3 : xbsIndex_r3/Slice  mode=Lower Bit Location + Width  nbits=16  bit1=0  base1=MSB of Input  bit0=16  base0=LSB of Input  boolean_output=off  explicit_period=off  period=1  dbl_ovrd=off
  slc_bitselect_4 : xbsIndex_r3/Slice  mode=Lower Bit Location + Width  nbits=16  bit1=0  base1=MSB of Input  bit0=24  base0=LSB of Input  boolean_output=off  explicit_period=off  period=1  dbl_ovrd=off
  slc_bitselect_5 : xbsIndex_r3/Slice  mode=Lower Bit Location + Width  nbits=16  bit1=0  base1=MSB of Input  bit0=32  base0=LSB of Input  boolean_output=off  explicit_period=off  period=1  dbl_ovrd=off
  slc_bitselect_6 : xbsIndex_r3/Slice  mode=Lower Bit Location + Width  nbits=16  bit1=0  base1=MSB of Input  bit0=40  base0=LSB of Input  boolean_output=off  explicit_period=off  period=1  dbl_ovrd=off
  slc_bitselect_7 : xbsIndex_r3/Slice  mode=Lower Bit Location + Width  nbits=16  bit1=0  base1=MSB of Input  bit0=48  base0=LSB of Input  boolean_output=off  explicit_period=off  period=1  dbl_ovrd=off
  data_out : Outport
  wires:
  slc_bitselect_1/1 -> mux_bitselect/2
  slc_bitselect_2/1 -> mux_bitselect/3
  slc_bitselect_3/1 -> mux_bitselect/4
  slc_bitselect_4/1 -> mux_bitselect/5
  data_in/1 -> reint_bp_0/1
  bitselect/1 -> mux_bitselect/1
  mux_bitselect/1 -> data_out/1
  reint_bp_0/1 -> slc_bitselect_3/1, slc_bitselect_4/1, slc_bitselect_5/1, slc_bitselect_6/1, slc_bitselect_7/1, slc_bitselect_2/1, slc_bitselect_1/1
  slc_bitselect_5/1 -> mux_bitselect/6
  slc_bitselect_7/1 -> mux_bitselect/8
  slc_bitselect_6/1 -> mux_bitselect/7

== system meat_1024pt_bee2_sign/unsigned_bitselect_4 ==
  bitselect : Inport  Port=1  LatchInput=off
  data_in : Inport  Port=2  LatchInput=off
  mux_bitselect : xbsIndex_r3/Mux  inputs=6  precision=Full  arith_type="Signed  (2's comp)"  n_bits=8  bin_pt=2  quantization=Truncate  overflow=Wrap  latency=1  explicit_period=off  period=1  en=off  dbl_ovrd=off  show_param=off  mux_type=off  use_rpm=off  gen_core=off
      settings: xl_area=[0, 0, 0, 0, 0, 0, 0]
  reint_bp_0 : xbsIndex_r3/Reinterpret  force_arith_type=on  arith_type=Unsigned  force_bin_pt=on  bin_pt=0  force_valid=on
  slc_bitselect_1 : xbsIndex_r3/Slice  mode=Lower Bit Location + Width  nbits=8  bit1=0  base1=MSB of Input  bit0=0  base0=LSB of Input  boolean_output=off  explicit_period=off  period=1  dbl_ovrd=off
  slc_bitselect_2 : xbsIndex_r3/Slice  mode=Lower Bit Location + Width  nbits=8  bit1=0  base1=MSB of Input  bit0=8  base0=LSB of Input  boolean_output=off  explicit_period=off  period=1  dbl_ovrd=off
  slc_bitselect_3 : xbsIndex_r3/Slice  mode=Lower Bit Location + Width  nbits=8  bit1=0  base1=MSB of Input  bit0=16  base0=LSB of Input  boolean_output=off  explicit_period=off  period=1  dbl_ovrd=off
  slc_bitselect_4 : xbsIndex_r3/Slice  mode=Lower Bit Location + Width  nbits=8  bit1=0  base1=MSB of Input  bit0=24  base0=LSB of Input  boolean_output=off  explicit_period=off  period=1  dbl_ovrd=off
  slc_bitselect_5 : xbsIndex_r3/Slice  mode=Lower Bit Location + Width  nbits=8  bit1=0  base1=MSB of Input  bit0=32  base0=LSB of Input  boolean_output=off  explicit_period=off  period=1  dbl_ovrd=off
  slc_bitselect_6 : xbsIndex_r3/Slice  mode=Lower Bit Location + Width  nbits=8  bit1=0  base1=MSB of Input  bit0=40  base0=LSB of Input  boolean_output=off  explicit_period=off  period=1  dbl_ovrd=off
  data_out : Outport
  wires:
  slc_bitselect_5/1 -> mux_bitselect/6
  slc_bitselect_6/1 -> mux_bitselect/7
  slc_bitselect_1/1 -> mux_bitselect/2
  slc_bitselect_2/1 -> mux_bitselect/3
  slc_bitselect_3/1 -> mux_bitselect/4
  slc_bitselect_4/1 -> mux_bitselect/5
  data_in/1 -> reint_bp_0/1
  bitselect/1 -> mux_bitselect/1
  mux_bitselect/1 -> data_out/1
  reint_bp_0/1 -> slc_bitselect_6/1, slc_bitselect_5/1, slc_bitselect_4/1, slc_bitselect_3/1, slc_bitselect_2/1, slc_bitselect_1/1

== system meat_1024pt_bee2_sign/unsigned_scale1 ==
  note: Unsigned, 18-bits, b.p. at 12
  note: Input unsigned 24-bits, b.p. at 23
  coeff : Inport  Orientation=down  Port=1  LatchInput=off
  data_in : Inport  Port=2  LatchInput=off
  Convert : xbsIndex_r3/Convert  arith_type=Unsigned  n_bits=32  bin_pt=31  quantization=Truncate  overflow=Wrap  latency=1  explicit_period=off  period=1  dbl_ovrd=off  show_param=off  inserted_by_tool=off  pipeline=off
      settings: xl_area=[0, 0, 0, 0, 0, 0, 0]
  mult_coeff_fft_real : xbsIndex_r3/Mult  precision=Full  arith_type="Signed  (2's comp)"  n_bits=24  bin_pt=23  quantization=Truncate  overflow=Wrap  latency=5  explicit_period=off  period=1  en=off  dbl_ovrd=off  show_param=on  mult_type=Parallel  oversample=2  use_embedded=on  pipeline=on  use_rpm=on  placement_style=Rectangular Shape  gen_core=off
      settings: xl_area=[0, 0, 0, 0, 0, 0, 0]
  data_out : Outport
  wires:
  mult_coeff_fft_real/1 -> Convert/1
  coeff/1 -> mult_coeff_fft_real/1
  data_in/1 -> mult_coeff_fft_real/2
  Convert/1 -> data_out/1

== system meat_1024pt_bee2_sign/unsigned_scale2 ==
  note: Input unsigned 24-bits, b.p. at 23
  note: Output unsigned 24-bits, b.p. at 23
  note: Unsigned, 18-bits, b.p. at 12
  coeff : Inport  Orientation=down  Port=1  LatchInput=off
  data_in : Inport  Port=2  LatchInput=off
  Convert : xbsIndex_r3/Convert  arith_type=Unsigned  n_bits=32  bin_pt=31  quantization=Truncate  overflow=Wrap  latency=1  explicit_period=off  period=1  dbl_ovrd=off  show_param=off  inserted_by_tool=off  pipeline=off
      settings: xl_area=[0, 0, 0, 0, 0, 0, 0]
  mult_coeff_fft_real : xbsIndex_r3/Mult  precision=Full  arith_type="Signed  (2's comp)"  n_bits=24  bin_pt=23  quantization=Truncate  overflow=Wrap  latency=5  explicit_period=off  period=1  en=off  dbl_ovrd=off  show_param=on  mult_type=Parallel  oversample=2  use_embedded=on  pipeline=on  use_rpm=on  placement_style=Rectangular Shape  gen_core=off
      settings: xl_area=[0, 0, 0, 0, 0, 0, 0]
  data_out : Outport
  wires:
  data_in/1 -> mult_coeff_fft_real/2
  coeff/1 -> mult_coeff_fft_real/1
  mult_coeff_fft_real/1 -> Convert/1
  Convert/1 -> data_out/1

== system meat_1024pt_bee2_sign/vacc ==
  note: The slice selects the upper bits of the
      | counter which represent the vector number.
  note: Acc Len is the total number of vectors accumulated minus one
      | Thus acc_len = 0 causes no accumulation, the data is passed through
  note: Valid goes high when dout
      | represents a valid accumulation
  note: ValidDelay should be equal to
      | Add Latency + Mux Latency to align the valid pulse with the output data.
  note: We want to generate a sync pulse that
      | will reset the counter right when the low bits
      | would roll over from veclen-1 to 0 so we need
      | to compare to veclen-2 to take into account
      | the latency in the comparator
  sync : Inport  Port=1  LatchInput=off
  din : Inport  Port=2  LatchInput=off
  acc_len : Inport  Port=3  LatchInput=off
  AND : xbsIndex_r3/Logical  logical_function=AND  inputs=2  precision=Full  arith_type=Unsigned  n_bits=8  bin_pt=2  align_bp=on  latency=0  explicit_period=off  period=1  en=off  dbl_ovrd=off  show_param=off
      settings: xl_area=[0, 0, 0, 0, 0, 0, 0]
  AccEnCompare : xbsIndex_r3/Relational  mode=a!=b  latency=1  explicit_period=off  period=1  en=off  dbl_ovrd=off  show_param=off
      settings: xl_area=[0, 0, 0, 0, 0, 0, 0]
  Counter : xbsIndex_r3/Counter  cnt_type=Free Running  n_bits=20  bin_pt=0  arith_type=Unsigned  start_count=0  cnt_to=Inf  cnt_by_val=1  operation=Up  explicit_period=on  period=1  load_pin=off  rst=on  en=off  dbl_ovrd=off  show_param=off  use_rpm=on  gen_core=off
      settings: xl_area=[0, 0, 0, 0, 0, 0, 0]
  Cram : Subsystem  AncestorBlock=gavrt_library/cram  mask(cram){num_slice=2}
      mask prompts: num_slice "Number of slices"
      mask help: Concatenates inputs together after forcing binary point to zero.
      mask init:
      | cram_init(gcb, ...
      |     'num_slice', num_slice);
  DinDelay : xbsIndex_r3/Delay  latency=2  reg_retiming=on  explicit_period=off  period=1  en=off  accept_only_valid=off  init_zero=on  dbl_ovrd=off  show_param=off
      settings: xl_area=[0, 0, 0, 0, 0, 0, 0]
  OR : xbsIndex_r3/Logical  logical_function=OR  inputs=2  precision=Full  arith_type=Unsigned  n_bits=8  bin_pt=2  align_bp=on  latency=0  explicit_period=off  period=1  en=off  dbl_ovrd=off  show_param=off
      settings: xl_area=[0, 0, 0, 0, 0, 0, 0]
  Slice : xbsIndex_r3/Slice  mode=Upper Bit Location + Width  nbits=10  bit1=0  base1=MSB of Input  bit0=0  base0=LSB of Input  boolean_output=off  explicit_period=off  period=1  dbl_ovrd=off
  SliceLow : xbsIndex_r3/Slice  mode=Lower Bit Location + Width  nbits=10  bit1=0  base1=MSB of Input  bit0=0  base0=LSB of Input  boolean_output=off  explicit_period=off  period=1  dbl_ovrd=off
  SyncCompare : xbsIndex_r3/Relational  mode=a=b  latency=1  explicit_period=off  period=1  en=off  dbl_ovrd=off  show_param=off
      settings: xl_area=[0, 0, 0, 0, 0, 0, 0]
  SyncConst : xbsIndex_r3/Constant  const=1022  equ=P=C  arith_type=Unsigned  n_bits=10  bin_pt=0  opselect=C  inp2=PCIN>>17  opr=+  inp1=P  carry=CIN  iostate=0  explicit_period=on  period=1  dbl_ovrd=off
  SyncDelay : xbsIndex_r3/Delay  latency=0  reg_retiming=off  explicit_period=off  period=1  en=off  accept_only_valid=off  init_zero=on  dbl_ovrd=off  show_param=off
      settings: xl_area=[0, 0, 0, 0, 0, 0, 0]
  Uncram : Subsystem  AncestorBlock=gavrt_library/uncram  mask(uncram){num_slice=2, slice_width=32, bin_pt=31, arith_type=1}
      mask prompts: num_slice "Number of slices"; slice_width "Slice Width"; bin_pt "Output Binary Point"; arith_type "Output Arithmetic Type (0=Unsigned, 1=Signed, 2=Boolean)"
      mask help: Takes a concatenated input and slices it up into even pieces and reinterprets them as signed fixed point numbers with a given binary point.
      mask init:
      | uncram_init(gcb, ...
      |     'num_slice', num_slice, ...
      |     'slice_width', slice_width, ...
      |     'bin_pt', bin_pt, ...
      |     'arith_type', arith_type);
      settings: AttributesFormatString=Fix_32_31
  ValidCompare : xbsIndex_r3/Relational  mode=a=b  latency=1  explicit_period=off  period=1  en=off  dbl_ovrd=off  show_param=off
      settings: xl_area=[0, 0, 0, 0, 0, 0, 0]
  ValidDelay : xbsIndex_r3/Delay  latency=3  reg_retiming=off  explicit_period=off  period=1  en=off  accept_only_valid=off  init_zero=on  dbl_ovrd=off  show_param=off
      settings: xl_area=[0, 0, 0, 0, 0, 0, 0]
  Zero : xbsIndex_r3/Constant  const=0  equ=P=C  arith_type=Unsigned  n_bits=8  bin_pt=0  opselect=C  inp2=PCIN>>17  opr=+  inp1=P  carry=CIN  iostate=0  explicit_period=on  period=1  dbl_ovrd=off
  vacc_core1 : Subsystem  AncestorBlock=gavrt_library/vacc_core  mask(vacc_core){veclen=1024, arith_type=1, out_bit_width=48, out_bin_pt=31, add_latency=2, bram_latency=2, mux_latency=1}
      mask prompts: veclen "Vector Length"; arith_type "Arithmetic Type (0=Unsigned, 1=Signed)"; out_bit_width "Output Bit Width"; out_bin_pt "Output Binary Point"; add_latency "Add Latency"; bram_latency "BRAM Latency"; mux_latency "Mux Latency"
      mask help:
      | Currently only Signed arithmetic supported
      | acc_en = 0 --> Load a vector (start a new accumulation)
      | acc_en = 1 --> Accumulate
      mask init:
      | vacc_core_init(gcb, ...
      |     'veclen', veclen, ...
      |     'arith_type', arith_type, ...
      |     'out_bit_width', out_bit_width, ...
      |     'out_bin_pt', out_bin_pt, ...
      |     'add_latency', add_latency, ...
      |     'bram_latency', bram_latency, ...
      |     'mux_latency', mux_latency);
  vacc_core2 : Subsystem  AncestorBlock=gavrt_library/vacc_core  mask(vacc_core){veclen=1024, arith_type=1, out_bit_width=48, out_bin_pt=31, add_latency=2, bram_latency=2, mux_latency=1}
      mask prompts: veclen "Vector Length"; arith_type "Arithmetic Type (0=Unsigned, 1=Signed)"; out_bit_width "Output Bit Width"; out_bin_pt "Output Binary Point"; add_latency "Add Latency"; bram_latency "BRAM Latency"; mux_latency "Mux Latency"
      mask help:
      | Currently only Signed arithmetic supported
      | acc_en = 0 --> Load a vector (start a new accumulation)
      | acc_en = 1 --> Accumulate
      mask init: same as meat_1024pt_bee2_sign/vacc/vacc_core1
  valid : Outport
  dout : Outport  Port=2
  wires:
  sync/1 -> SyncDelay/1
  SyncDelay/1 -> OR/1
  [valid] -> AND/1
  AND/1 -> OR/2
  OR/1 -> Counter/1
  Counter/1 -> [count], Slice/1
  [count] -> SliceLow/1
  SliceLow/1 -> SyncCompare/1
  SyncConst/1 -> SyncCompare/2
  SyncCompare/1 -> AND/2
  ValidCompare/1 -> [valid], ValidDelay/1
  acc_len/1 -> ValidCompare/1
  Slice/1 -> ValidCompare/2, AccEnCompare/1
  Zero/1 -> AccEnCompare/2
  ValidDelay/1 -> valid/1
  din/1 -> DinDelay/1
  DinDelay/1 -> Uncram/1(In)
  Cram/1(Out) -> dout/1
  Uncram/1(Out1) -> vacc_core1/1(din)
  AccEnCompare/1 -> vacc_core1/2(acc_en), vacc_core2/2(acc_en)
  vacc_core1/1(dout) -> Cram/1(In1)
  Uncram/2(Out2) -> vacc_core2/1(din)
  vacc_core2/1(dout) -> Cram/2(In2)

== system meat_1024pt_bee2_sign/vacc1 ==
  note: We want to generate a sync pulse that
      | will reset the counter right when the low bits
      | would roll over from veclen-1 to 0 so we need
      | to compare to veclen-2 to take into account
      | the latency in the comparator
  note: ValidDelay should be equal to
      | Add Latency + Mux Latency to align the valid pulse with the output data.
  note: Valid goes high when dout
      | represents a valid accumulation
  note: Acc Len is the total number of vectors accumulated minus one
      | Thus acc_len = 0 causes no accumulation, the data is passed through
  note: The slice selects the upper bits of the
      | counter which represent the vector number.
  sync : Inport  Port=1  LatchInput=off
  din : Inport  Port=2  LatchInput=off
  acc_len : Inport  Port=3  LatchInput=off
  AND : xbsIndex_r3/Logical  logical_function=AND  inputs=2  precision=Full  arith_type=Unsigned  n_bits=8  bin_pt=2  align_bp=on  latency=0  explicit_period=off  period=1  en=off  dbl_ovrd=off  show_param=off
      settings: xl_area=[0, 0, 0, 0, 0, 0, 0]
  AccEnCompare : xbsIndex_r3/Relational  mode=a!=b  latency=1  explicit_period=off  period=1  en=off  dbl_ovrd=off  show_param=off
      settings: xl_area=[0, 0, 0, 0, 0, 0, 0]
  Counter : xbsIndex_r3/Counter  cnt_type=Free Running  n_bits=20  bin_pt=0  arith_type=Unsigned  start_count=0  cnt_to=Inf  cnt_by_val=1  operation=Up  explicit_period=on  period=1  load_pin=off  rst=on  en=off  dbl_ovrd=off  show_param=off  use_rpm=on  gen_core=off
      settings: xl_area=[0, 0, 0, 0, 0, 0, 0]
  Cram : Subsystem  AncestorBlock=gavrt_library/cram  mask(cram){num_slice=2}
      mask prompts: num_slice "Number of slices"
      mask help: Concatenates inputs together after forcing binary point to zero.
      mask init:
      | cram_init(gcb, ...
      |     'num_slice', num_slice);
  DinDelay : xbsIndex_r3/Delay  latency=2  reg_retiming=on  explicit_period=off  period=1  en=off  accept_only_valid=off  init_zero=on  dbl_ovrd=off  show_param=off
      settings: xl_area=[0, 0, 0, 0, 0, 0, 0]
  OR : xbsIndex_r3/Logical  logical_function=OR  inputs=2  precision=Full  arith_type=Unsigned  n_bits=8  bin_pt=2  align_bp=on  latency=0  explicit_period=off  period=1  en=off  dbl_ovrd=off  show_param=off
      settings: xl_area=[0, 0, 0, 0, 0, 0, 0]
  Slice : xbsIndex_r3/Slice  mode=Upper Bit Location + Width  nbits=10  bit1=0  base1=MSB of Input  bit0=0  base0=LSB of Input  boolean_output=off  explicit_period=off  period=1  dbl_ovrd=off
  SliceLow : xbsIndex_r3/Slice  mode=Lower Bit Location + Width  nbits=10  bit1=0  base1=MSB of Input  bit0=0  base0=LSB of Input  boolean_output=off  explicit_period=off  period=1  dbl_ovrd=off
  SyncCompare : xbsIndex_r3/Relational  mode=a=b  latency=1  explicit_period=off  period=1  en=off  dbl_ovrd=off  show_param=off
      settings: xl_area=[0, 0, 0, 0, 0, 0, 0]
  SyncConst : xbsIndex_r3/Constant  const=1022  equ=P=C  arith_type=Unsigned  n_bits=10  bin_pt=0  opselect=C  inp2=PCIN>>17  opr=+  inp1=P  carry=CIN  iostate=0  explicit_period=on  period=1  dbl_ovrd=off
  SyncDelay : xbsIndex_r3/Delay  latency=0  reg_retiming=off  explicit_period=off  period=1  en=off  accept_only_valid=off  init_zero=on  dbl_ovrd=off  show_param=off
      settings: xl_area=[0, 0, 0, 0, 0, 0, 0]
  Uncram : Subsystem  AncestorBlock=gavrt_library/uncram  mask(uncram){num_slice=2, slice_width=32, bin_pt=31, arith_type=0}
      mask prompts: num_slice "Number of slices"; slice_width "Slice Width"; bin_pt "Output Binary Point"; arith_type "Output Arithmetic Type (0=Unsigned, 1=Signed, 2=Boolean)"
      mask help: Takes a concatenated input and slices it up into even pieces and reinterprets them as signed fixed point numbers with a given binary point.
      mask init:
      | uncram_init(gcb, ...
      |     'num_slice', num_slice, ...
      |     'slice_width', slice_width, ...
      |     'bin_pt', bin_pt, ...
      |     'arith_type', arith_type);
      settings: AttributesFormatString=UFix_32_31
  ValidCompare : xbsIndex_r3/Relational  mode=a=b  latency=1  explicit_period=off  period=1  en=off  dbl_ovrd=off  show_param=off
      settings: xl_area=[0, 0, 0, 0, 0, 0, 0]
  ValidDelay : xbsIndex_r3/Delay  latency=3  reg_retiming=off  explicit_period=off  period=1  en=off  accept_only_valid=off  init_zero=on  dbl_ovrd=off  show_param=off
      settings: xl_area=[0, 0, 0, 0, 0, 0, 0]
  Zero : xbsIndex_r3/Constant  const=0  equ=P=C  arith_type=Unsigned  n_bits=8  bin_pt=0  opselect=C  inp2=PCIN>>17  opr=+  inp1=P  carry=CIN  iostate=0  explicit_period=on  period=1  dbl_ovrd=off
  vacc_core1 : Subsystem  AncestorBlock=gavrt_library/vacc_core  mask(vacc_core){veclen=1024, arith_type=0, out_bit_width=48, out_bin_pt=31, add_latency=2, bram_latency=2, mux_latency=1}
      mask prompts: veclen "Vector Length"; arith_type "Arithmetic Type (0=Unsigned, 1=Signed)"; out_bit_width "Output Bit Width"; out_bin_pt "Output Binary Point"; add_latency "Add Latency"; bram_latency "BRAM Latency"; mux_latency "Mux Latency"
      mask help:
      | Currently only Signed arithmetic supported
      | acc_en = 0 --> Load a vector (start a new accumulation)
      | acc_en = 1 --> Accumulate
      mask init: same as meat_1024pt_bee2_sign/vacc/vacc_core1
  vacc_core2 : Subsystem  AncestorBlock=gavrt_library/vacc_core  mask(vacc_core){veclen=1024, arith_type=0, out_bit_width=48, out_bin_pt=31, add_latency=2, bram_latency=2, mux_latency=1}
      mask prompts: veclen "Vector Length"; arith_type "Arithmetic Type (0=Unsigned, 1=Signed)"; out_bit_width "Output Bit Width"; out_bin_pt "Output Binary Point"; add_latency "Add Latency"; bram_latency "BRAM Latency"; mux_latency "Mux Latency"
      mask help:
      | Currently only Signed arithmetic supported
      | acc_en = 0 --> Load a vector (start a new accumulation)
      | acc_en = 1 --> Accumulate
      mask init: same as meat_1024pt_bee2_sign/vacc/vacc_core1
  valid : Outport
  dout : Outport  Port=2
  wires:
  sync/1 -> SyncDelay/1
  SyncDelay/1 -> OR/1
  [valid] -> AND/1
  AND/1 -> OR/2
  OR/1 -> Counter/1
  Counter/1 -> [count], Slice/1
  [count] -> SliceLow/1
  SliceLow/1 -> SyncCompare/1
  SyncConst/1 -> SyncCompare/2
  SyncCompare/1 -> AND/2
  ValidCompare/1 -> [valid], ValidDelay/1
  acc_len/1 -> ValidCompare/1
  Slice/1 -> ValidCompare/2, AccEnCompare/1
  Zero/1 -> AccEnCompare/2
  ValidDelay/1 -> valid/1
  din/1 -> DinDelay/1
  DinDelay/1 -> Uncram/1(In)
  Cram/1(Out) -> dout/1
  Uncram/1(Out1) -> vacc_core1/1(din)
  AccEnCompare/1 -> vacc_core1/2(acc_en), vacc_core2/2(acc_en)
  vacc_core1/1(dout) -> Cram/1(In1)
  Uncram/2(Out2) -> vacc_core2/1(din)
  vacc_core2/1(dout) -> Cram/2(In2)
